simulink model "svpwm"  (R2021b)
settings: Solver=FixedStepAuto  StartTime=0.0  StopTime=10  FixedStep=1e-4  RelTol=1e-3
values from neighbouring files (symbols this model uses):
  flux = 0.016884    [svpwm.sldd]
  Pn = 4.0    [svpwm.sldd]
undefined symbols (not defined in the file or in its folder): Udc
libraries: mcbplantlib x1, autolibpmsmexterior x1
settings Model: DataDictionary=SVPWM.sldd  Creator=ssc  LastModifiedBy=ssc
settings OptimizationCC: DefaultParameterBehavior=Inlined  UseDivisionForNetSlopeComputation=on  GainParamInheritBuiltInType=on  UseFloatMulNetSlope=on  InlineInvariantSignals=on  PassReuseOutputArgsAs=Individual arguments  ZeroExternalMemoryAtStartup=off  ZeroInternalMemoryAtStartup=off  NoFixptDivByZeroProtection=on  EfficientFloat2IntCast=on  LifeSpan=1  OptimizeBlockOrder=speed  DifferentSizesBufferReuse=on  EfficientTunableParamExpr=on
settings DebuggingCC: ParameterTunabilityLossMsg=error
settings HardwareCC: ProdBitPerPointer=32  ProdBitPerSizeT=32  ProdBitPerPtrDiffT=32  ProdLargestAtomicInteger=Long  ProdLargestAtomicFloat=Double  ProdWordSize=32  ProdLongLongMode=on  ProdHWDeviceType=ARM Compatible->ARM Cortex-M
settings SFSimCC: MATLABDynamicMemAlloc=off
settings RTWCC: Description=Embedded Coder  SystemTargetFile=ert.tlc  TemplateMakefile=ert_default_tmf  GenerateReport=on  LaunchReport=on
settings CodeAppCC: ForceParamTrailComments=on  IgnoreCustomStorageClasses=off  OperatorAnnotations=on  SimulinkDataObjDesc=on  SFDataObjDesc=on  CustomSymbolStrGlobalVar=rt$N$M  CustomSymbolStrType=$N$M  CustomSymbolStrFcn=$N$M$F  CustomSymbolStrMacro=$N$M  InsertBlockDesc=on
settings ERTTargetCC: TargetLangStandard=C99 (ISO)  CodeReplacementLibrary=ARM Cortex-M  GenerateSampleERTMain=on  IncludeMdlTerminateFcn=off  CombineSignalStateStructs=on  SupportAbsoluteTime=off  SupportNonFinite=off  SupportComplex=off  InlinedParameterPlacement=NonHierarchical  ERTCustomFileTemplate=example_file_process.tlc  ERTFilePackagingFormat=CompactWithDataFile

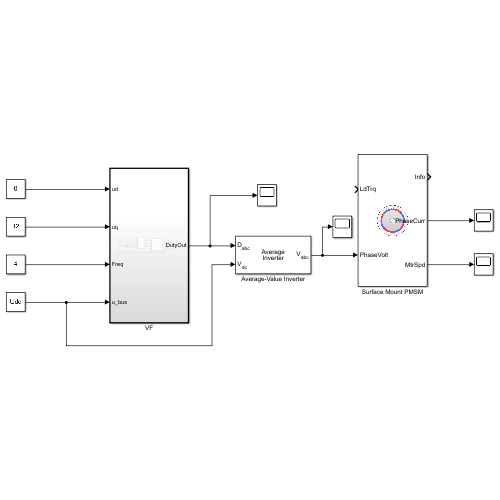
[thumbnail: Simulink's stored preview of the top-level diagram]
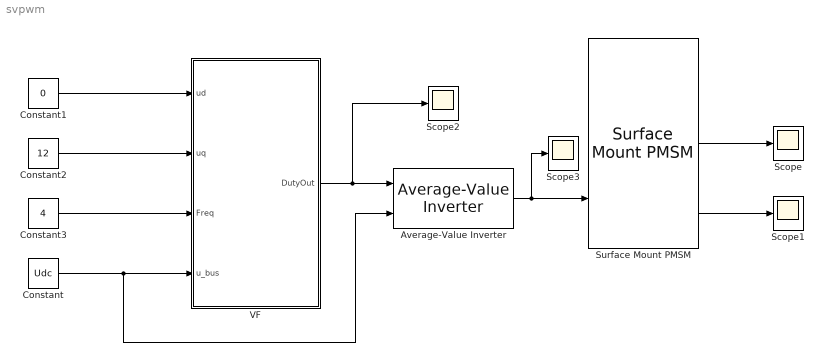
== system svpwm ==
  Average-Value Inverter : mcbplantlib/Average-Value Inverter
  Constant : Constant  Value=Udc
  Constant1 : Constant  Value=0
  Constant2 : Constant  Value=12
  Constant3 : Constant  Value=4
  Scope{,1..3} (4 alike) : Scope
  Surface Mount PMSM : autolibpmsmexterior/Surface Mount PMSM  port_config=Torque  sim_type=Continuous  Ts=0.001  P=Pn  Rs=Rs  Ldq_=L  KConstText=Permanent flux linkage constant (lambda_pm):  lambda_pm=flux  Ke=159.9771  Kt=1.323  mechanical=[75e-6,8e-5,0]  idq0=[0 0]  theta_init=0  omega_init=0  KConst=flux  lambda_pm_calc=flux  RefBlkName='autolibpmsmexterior/Surface Mount PMSM'  aMode=5  Ldq="[0.0017      0.0017]"
      settings: SourceProductBaseCode=PW,DR,MT,UV,VE
  VF : Subsystem  TreatAsAtomicUnit=on
  wires:
  VF/1(DutyOut) -> Scope2/1, Average-Value Inverter/1
  Constant/1 -> Average-Value Inverter/2, VF/4(u_bus)
  Constant2/1 -> VF/2(uq)
  Constant1/1 -> VF/1(ud)
  Constant3/1 -> VF/3(Freq)
  Average-Value Inverter/1 -> Scope3/1, Surface Mount PMSM/2
  Surface Mount PMSM/2 -> Scope/1
  Surface Mount PMSM/3 -> Scope1/1

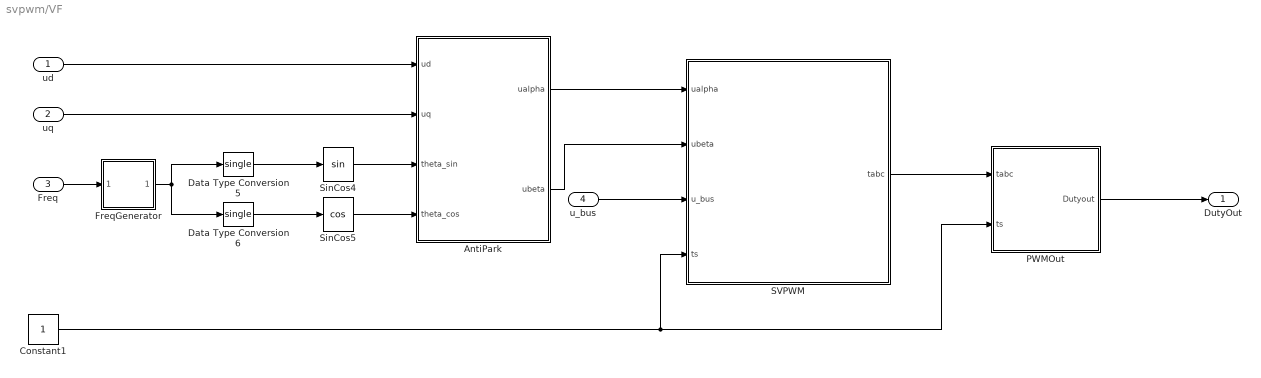
== system svpwm/VF ==
  ud : Inport
  uq : Inport  Port=2
  Freq : Inport  Port=3
  u_bus : Inport  Port=4
  AntiPark : Subsystem
  Constant1 : Constant
  Data Type Conversion5 : DataTypeConversion  OutDataTypeStr=single
  Data Type Conversion6 : DataTypeConversion  OutDataTypeStr=single
  FreqGenerator : Subsystem
  PWMOut : Subsystem
  SVPWM : Subsystem
  SinCos4 : Trigonometry
  SinCos5 : Trigonometry  Operator=cos
  DutyOut : Outport
  wires:
  FreqGenerator/1(Theta) -> Data Type Conversion6/1, Data Type Conversion5/1
  Constant1/1 -> PWMOut/2(ts), SVPWM/4(ts)
  SVPWM/1(tabc) -> PWMOut/1(tabc)
  SinCos5/1 -> AntiPark/4(theta_cos)
  SinCos4/1 -> AntiPark/3(theta_sin)
  Data Type Conversion5/1 -> SinCos4/1
  ud/1 -> AntiPark/1(ud)
  Data Type Conversion6/1 -> SinCos5/1
  u_bus/1 -> SVPWM/3(u_bus)
  uq/1 -> AntiPark/2(uq)
  PWMOut/1(Dutyout) -> DutyOut/1
  Freq/1 -> FreqGenerator/1(Freq)
  AntiPark/1(ualpha) -> SVPWM/1(ualpha)
  AntiPark/2(ubeta) -> SVPWM/2(ubeta)

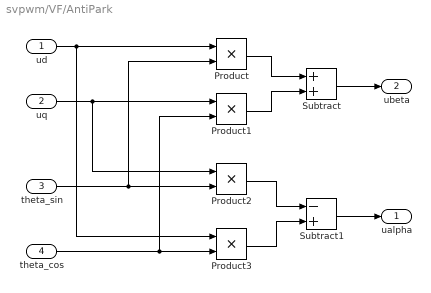
== system svpwm/VF/AntiPark ==
  ud : Inport
  uq : Inport  Port=2
  theta_sin : Inport  Port=3
  theta_cos : Inport  Port=4
  Product{,1..3} (4 alike) : Product
  Subtract : Sum
  Subtract1 : Sum  Inputs=-+
  ualpha : Outport
  ubeta : Outport  Port=2
  wires:
  ud/1 -> Product/1, Product3/1
  theta_sin/1 -> Product2/2, Product/2
  uq/1 -> Product1/1, Product2/1
  theta_cos/1 -> Product3/2, Product1/2
  Product/1 -> Subtract/1
  Product1/1 -> Subtract/2
  Product2/1 -> Subtract1/1
  Product3/1 -> Subtract1/2
  Subtract/1 -> ubeta/1
  Subtract1/1 -> ualpha/1

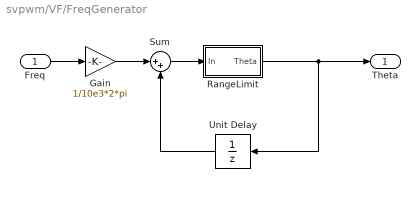
== system svpwm/VF/FreqGenerator ==
  Freq : Inport
  Gain : Gain  Gain=1/10e3*2*pi  OutDataTypeStr=single
  RangeLimit : Subsystem
  Sum : Sum  Inputs=|++  OutDataTypeStr=Inherit: Same as first input
  Unit Delay : UnitDelay  SampleTime=-1  HasFrameUpgradeWarning=on
  Theta : Outport
  wires:
  Freq/1 -> Gain/1
  RangeLimit/1(Theta) -> Theta/1, Unit Delay/1
  Gain/1 -> Sum/1
  Sum/1 -> RangeLimit/1(In)
  Unit Delay/1 -> Sum/2

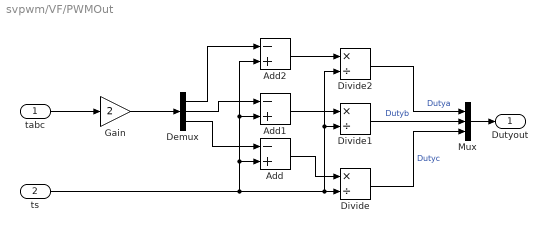
== system svpwm/VF/PWMOut ==
  tabc : Inport
  ts : Inport  Port=2
  Add : Sum  Inputs=-+
  Add1 : Sum  Inputs=-+
  Add2 : Sum  Inputs=-+
  Demux : Demux  Outputs=3
  Divide : Product  Inputs=*/
  Divide1 : Product  Inputs=*/
  Divide2 : Product  Inputs=*/
  Gain : Gain  Gain=2
  Mux : Mux  Inputs=3
  Dutyout : Outport
  wires:
  tabc/1 -> Gain/1
  Gain/1 -> Demux/1
  ts/1 -> Add1/2, Add2/2, Add/2, Divide2/2, Divide1/2, Divide/2
  Demux/3 -> Add/1
  Add/1 -> Divide/1
  Divide/1 -> Mux/3  "Dutyc"
  Demux/1 -> Add2/1
  Add1/1 -> Divide1/1
  Add2/1 -> Divide2/1
  Demux/2 -> Add1/1
  Divide1/1 -> Mux/2  "Dutyb"
  Divide2/1 -> Mux/1  "Dutya"
  Mux/1 -> Dutyout/1

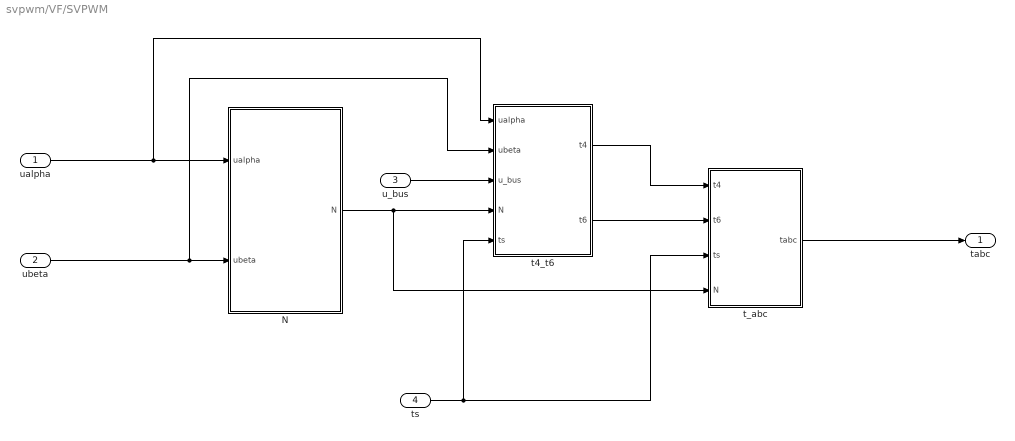
== system svpwm/VF/SVPWM ==
  ualpha : Inport
  ubeta : Inport  Port=2
  u_bus : Inport  Port=3
  ts : Inport  Port=4
  N : Subsystem
  t4_t6 : Subsystem
  t_abc : Subsystem
  tabc : Outport
  wires:
  ubeta/1 -> t4_t6/2(ubeta), N/2(ubeta)
  t4_t6/1(t4) -> t_abc/1(t4)
  N/1(N) -> t_abc/4(N), t4_t6/4(N)
  ualpha/1 -> t4_t6/1(ualpha), N/1(ualpha)
  t4_t6/2(t6) -> t_abc/2(t6)
  u_bus/1 -> t4_t6/3(u_bus)
  ts/1 -> t_abc/3(ts), t4_t6/5(ts)
  t_abc/1(tabc) -> tabc/1

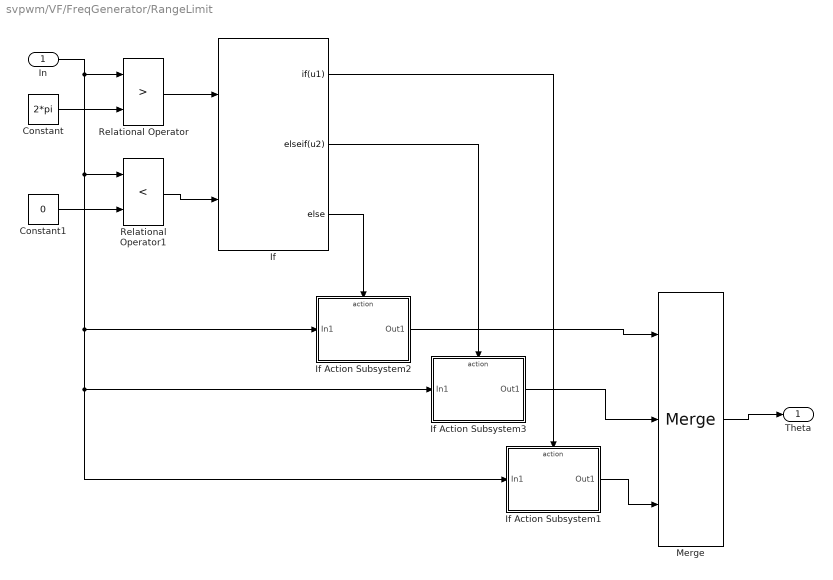
== system svpwm/VF/FreqGenerator/RangeLimit ==
  In : Inport
  Constant : Constant  Value=2*pi  OutDataTypeStr=single  SampleTime=-1
  Constant1 : Constant  Value=0  OutDataTypeStr=single  SampleTime=-1
  If : If  NumInputs=2  IfExpression=u1  ElseIfExpressions=u2
  If Action Subsystem1 : Subsystem  TreatAsAtomicUnit=on
  If Action Subsystem2 : Subsystem  TreatAsAtomicUnit=on
  If Action Subsystem3 : Subsystem  TreatAsAtomicUnit=on
  Merge : Merge  Inputs=3
  Relational Operator : RelationalOperator  Operator=>  OutDataTypeStr=boolean  RndMeth=Simplest
  Relational Operator1 : RelationalOperator  Operator=<  OutDataTypeStr=boolean  RndMeth=Simplest
  Theta : Outport
  wires:
  Relational Operator/1 -> If/1
  Constant/1 -> Relational Operator/2
  In/1 -> Relational Operator1/1, If Action Subsystem2/1(In1), If Action Subsystem3/1(In1), If Action Subsystem1/1(In1), Relational Operator/1
  Merge/1 -> Theta/1
  If/3 -> If Action Subsystem2/Action
  If/1 -> If Action Subsystem1/Action
  If Action Subsystem2/1(Out1) -> Merge/1
  Constant1/1 -> Relational Operator1/2
  Relational Operator1/1 -> If/2
  If/2 -> If Action Subsystem3/Action
  If Action Subsystem1/1(Out1) -> Merge/3
  If Action Subsystem3/1(Out1) -> Merge/2

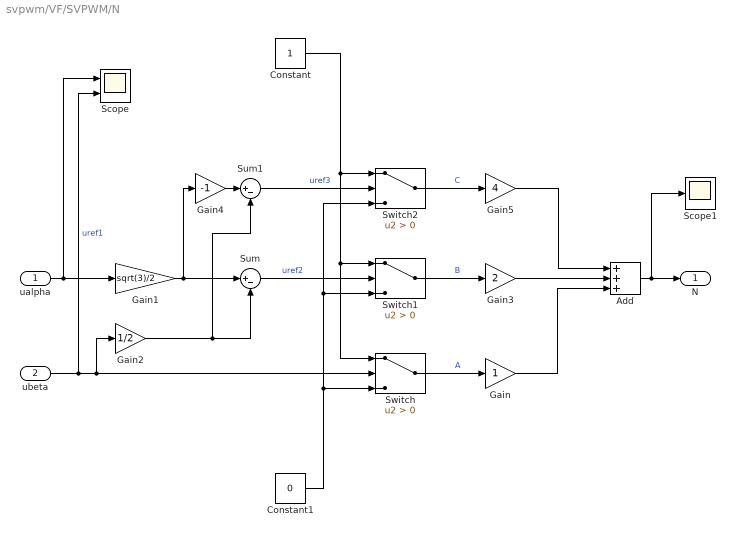
== system svpwm/VF/SVPWM/N ==
  ualpha : Inport
  ubeta : Inport  Port=2
  Add : Sum  Inputs=+++
  Constant : Constant  OutDataTypeStr=single
  Constant1 : Constant  Value=0  OutDataTypeStr=single
  Gain : Gain
  Gain1 : Gain  Gain=sqrt(3)/2
  Gain2 : Gain  Gain=1/2
  Gain3 : Gain  Gain=2
  Gain4 : Gain  Gain=-1
  Gain5 : Gain  Gain=4
  Scope : Scope  NumInputPorts=2
  Scope1 : Scope
  Sum : Sum  Inputs=|+-
  Sum1 : Sum  Inputs=|+-
  Switch : Switch  Criteria=u2 > Threshold
  Switch1 : Switch  Criteria=u2 > Threshold
  Switch2 : Switch  Criteria=u2 > Threshold
  N : Outport
  wires:
  ualpha/1 -> Gain1/1, Scope/1
  ubeta/1 -> Switch/2, Gain2/1, Scope/2  "uref1"
  Constant/1 -> Switch2/1, Switch1/1, Switch/1
  Constant1/1 -> Switch2/3, Switch1/3, Switch/3
  Switch/1 -> Gain/1  "A"
  Gain1/1 -> Gain4/1, Sum/1
  Gain2/1 -> Sum1/2, Sum/2
  Sum/1 -> Switch1/2  "uref2"
  Switch1/1 -> Gain3/1  "B"
  Gain4/1 -> Sum1/1
  Sum1/1 -> Switch2/2  "uref3"
  Switch2/1 -> Gain5/1  "C"
  Gain3/1 -> Add/2
  Add/1 -> Scope1/1, N/1
  Gain/1 -> Add/3
  Gain5/1 -> Add/1

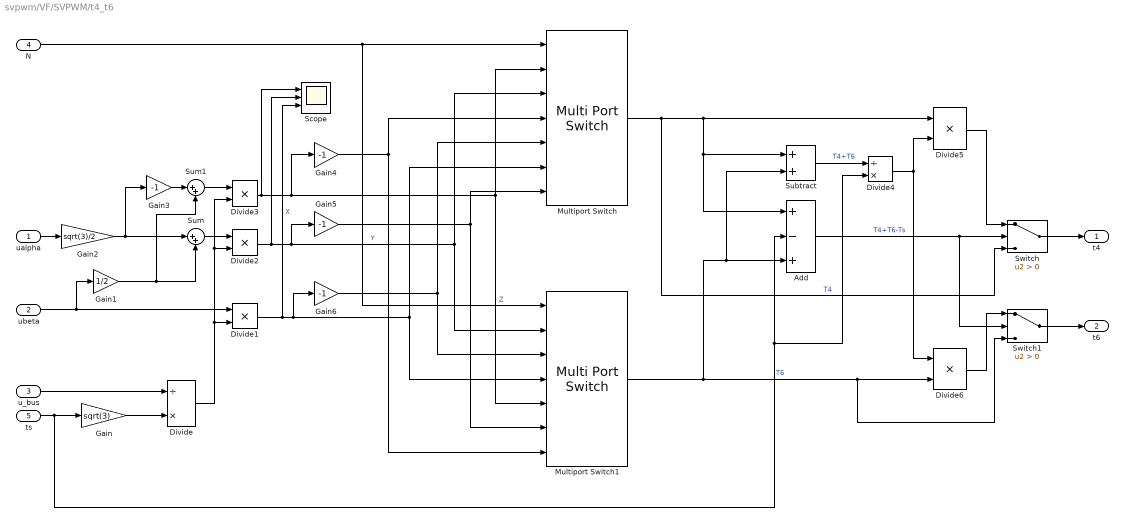
== system svpwm/VF/SVPWM/t4_t6 ==
  ualpha : Inport
  ubeta : Inport  Port=2
  u_bus : Inport  Port=3
  N : Inport  Port=4
  ts : Inport  Port=5
  Add : Sum  Inputs=+-+
  Divide : Product  Inputs=/*
  Divide{1..3,5..6} (5 alike) : Product  Inputs=**
  Divide4 : Product  Inputs=/*
  Gain : Gain  Gain=sqrt(3)
  Gain1 : Gain  Gain=1/2
  Gain2 : Gain  Gain=sqrt(3)/2
  Gain{3..6} (4 alike) : Gain  Gain=-1
  Multiport Switch : MultiPortSwitch  Inputs=6
  Multiport Switch1 : MultiPortSwitch  Inputs=6
  Scope : Scope  NumInputPorts=3
  Subtract : Sum
  Sum : Sum  Inputs=|++
  Sum1 : Sum  Inputs=|++
  Switch : Switch  Criteria=u2 > Threshold
  Switch1 : Switch  Criteria=u2 > Threshold
  t4 : Outport
  t6 : Outport  Port=2
  wires:
  ts/1 -> Gain/1, Divide4/2, Add/2
  u_bus/1 -> Divide/1
  Gain/1 -> Divide/2
  ubeta/1 -> Gain1/1, Divide1/1
  Divide/1 -> Divide3/2, Divide2/2, Divide1/2
  Divide1/1 -> Scope/3, Multiport Switch1/4, Multiport Switch/6, Gain6/1  "X"
  ualpha/1 -> Gain2/1
  Gain1/1 -> Sum1/2, Sum/2
  Gain2/1 -> Gain3/1, Sum/1
  Sum/1 -> Divide2/1
  Divide2/1 -> Scope/2, Multiport Switch1/2, Multiport Switch/3, Gain5/1  "Y"
  Gain3/1 -> Sum1/1
  Sum1/1 -> Divide3/1
  Divide3/1 -> Scope/1, Gain4/1, Multiport Switch1/5, Multiport Switch/2  "Z"
  N/1 -> Multiport Switch1/1, Multiport Switch/1
  Multiport Switch/1 -> Switch/3, Divide5/1, Subtract/1, Add/1  "T4"
  Gain6/1 -> Multiport Switch1/3, Multiport Switch/5
  Gain4/1 -> Multiport Switch1/7, Multiport Switch/4
  Gain5/1 -> Multiport Switch1/6, Multiport Switch/7
  Add/1 -> Switch1/2, Switch/2  "T4+T6-Ts"
  Multiport Switch1/1 -> Switch1/3, Divide6/2, Subtract/2, Add/3  "T6"
  Subtract/1 -> Divide4/1  "T4+T6"
  Divide4/1 -> Divide5/2, Divide6/1
  Divide5/1 -> Switch/1
  Divide6/1 -> Switch1/1
  Switch/1 -> t4/1
  Switch1/1 -> t6/1

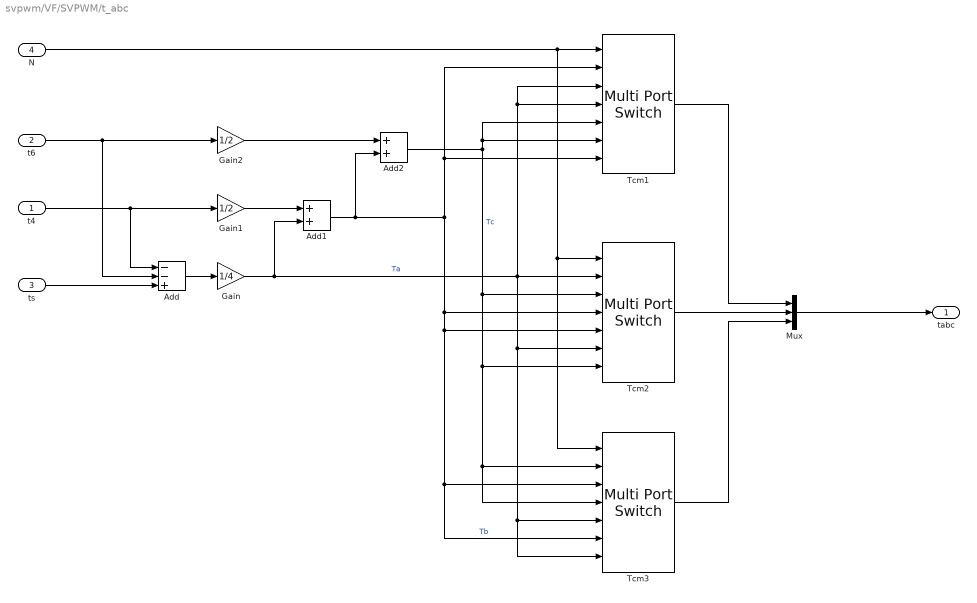
== system svpwm/VF/SVPWM/t_abc ==
  t4 : Inport
  t6 : Inport  Port=2
  ts : Inport  Port=3
  N : Inport  Port=4
  Add : Sum  Inputs=--+
  Add1 : Sum
  Add2 : Sum
  Gain : Gain  Gain=1/4
  Gain1 : Gain  Gain=1/2
  Gain2 : Gain  Gain=1/2
  Mux : Mux  Inputs=3
  "Tcm1 " : MultiPortSwitch  Inputs=6
  Tcm2 : MultiPortSwitch  Inputs=6
  Tcm3 : MultiPortSwitch  Inputs=6
  tabc : Outport
  wires:
  ts/1 -> Add/3
  t6/1 -> Add/2, Gain2/1
  t4/1 -> Add/1, Gain1/1
  Add/1 -> Gain/1
  Gain/1 -> Tcm2/6, Tcm3/7, Tcm3/5, "Tcm1 "/4, "Tcm1 "/3, Tcm2/2, Add1/2  "Ta"
  Gain1/1 -> Add1/1
  Gain2/1 -> Add2/1
  Add1/1 -> Add2/2, "Tcm1 "/7, "Tcm1 "/2, Tcm2/4, Tcm3/6, Tcm3/3, Tcm2/5  "Tb"
  N/1 -> Tcm3/1, Tcm2/1, "Tcm1 "/1
  Add2/1 -> "Tcm1 "/6, "Tcm1 "/5, Tcm3/4, Tcm3/2, Tcm2/7, Tcm2/3  "Tc"
  "Tcm1 "/1 -> Mux/1
  Tcm3/1 -> Mux/3
  Tcm2/1 -> Mux/2
  Mux/1 -> tabc/1

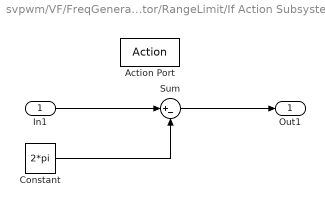
== system svpwm/VF/FreqGenerator/RangeLimit/If Action Subsystem1 ==
  In1 : Inport
  Action Port : ActionPort  ActionPortLabel=if(u1)
  Constant : Constant  Value=2*pi  OutDataTypeStr=single  SampleTime=-1
  Sum : Sum  Inputs=|+-
  Out1 : Outport
  wires:
  In1/1 -> Sum/1
  Constant/1 -> Sum/2
  Sum/1 -> Out1/1

== system svpwm/VF/FreqGenerator/RangeLimit/If Action Subsystem2 ==
  In1 : Inport
  Action Port : ActionPort  ActionPortLabel=else
  Out1 : Outport
  wires:
  In1/1 -> Out1/1

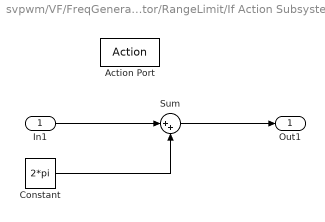
== system svpwm/VF/FreqGenerator/RangeLimit/If Action Subsystem3 ==
  In1 : Inport
  Action Port : ActionPort  ActionPortLabel=elseif(u2)
  Constant : Constant  Value=2*pi  OutDataTypeStr=single  SampleTime=-1
  Sum : Sum  Inputs=|++
  Out1 : Outport
  wires:
  Constant/1 -> Sum/2
  In1/1 -> Sum/1
  Sum/1 -> Out1/1
